simulink model "am_sys1"  (Simulink 3.00)
settings: Solver=ode45  StartTime=0.0  StopTime=999999  MaxStep=0.005  RelTol=1e-3  AbsTol=1e-3
settings Model: SaveTime=off  SaveOutput=off

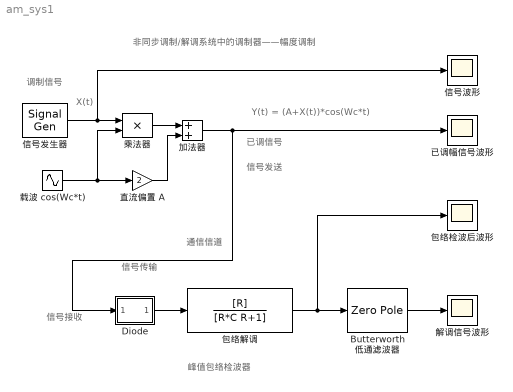
== system am_sys1 ==
  note: 峰值包络检波器
  note: 调制信号
  note: X(t)
  note: Y(t) = (A+X(t))*cos(Wc*t)
  note: 已调信号
  note: 信号发送
  note: 通信信道
  note: 信号传输
  note: 信号接收
  note: 非同步调制/解调系统中的调制器——幅度调制
  Butterworth 低通滤波器 : ZeroPole  Zeros=z  Poles=p  Gain=k  mask(buttap){@1=5*2*pi, @2=4}
      mask prompts: @1 "Cutoff frequency (rad/sec)"; @2 "Order"
      mask help:
      | Analog Butterworth low pass filter.
      |
      | (Requires Signal Processing Toolbox)
      mask init:
      | [z,p,k]=buttap(@2); z=@1*z; p=@1*p; k=real(prod(-p)); [num,den]=zp2tf(z,p,k); w=logspace(log10(@1/10),log10(10*@1),20); h=freqs(num,den,w);
      mask Help: Butterworth low pass filter using MATLAB's butter command.
      mask Display: plot(20*log10(w),20*log10(abs(h)))
  Diode : Subsystem
      mask Type: 二极管
      mask Description: 二极管
      mask Display: plot([0 2 2 2],[0 0 2 -2],[2 4],[2 0],[2 4],[-2 0],[4 4 4 6],[-2 2 0 0]);
  包络检波后波形 : Scope
      settings: TimeRange=1.000000  YMin=-1  YMax=1  SaveToWorkspace=off  SaveName=ScopeData  DataFormat=Matrix
  包络解调 : TransferFcn  Numerator=[R]  Denominator=[R*C R+1]  mask(单元6){@1=1, @2=0.1}
      mask prompts: @1 "电阻值（欧）："; @2 "电容值（法）："
      mask help: 单元6
      mask init:
      | R=@1;C=@2;
      mask Display: plot([0 15],[2 2],[8 8 6 10],[2 0 0 0],[6 10],[-1 -1],[8 8 7 9],[-1 -4 -4 -4],[12.5 12.5 12 13],[2 1 1 1],[12 12],[1 -3],[13 13],[1 -3],[12 13 12.5 12.5],[-3 -3 -3 -4],[12 13],[-4 -4]);
  乘法器 : Product  Inputs=2  SaturateOnIntegerOverflow=on
      mask Type: 乘法器
      mask Description: 乘法器
      mask Display: plot([0 1],[1 0],[0 1],[0 1]);
  加法器 : Sum  Inputs=++  SaturateOnIntegerOverflow=on
  解调信号波形 : Scope
      settings: TimeRange=1.000000  YMin=-0.5  YMax=0.5  SaveToWorkspace=off  SaveName=ScopeData  DataFormat=Matrix
  信号波形 : Scope
      settings: TimeRange=1.000000  YMin=-3  YMax=3  SaveToWorkspace=off  SaveName=ScopeData  DataFormat=Matrix
  信号发生器 : SignalGenerator  WaveForm=sine  Amplitude=1.000000  Frequency=30.000000  Units=rad/sec
  已调幅信号波形 : Scope
      settings: TimeRange=1.000000  YMin=-3  YMax=3  SaveToWorkspace=off  SaveName=ScopeData  DataFormat=Matrix
  载波 cos(Wc*t) : Sin  Amplitude=1  Frequency=F*2*pi  Phase=0  SampleTime=0.005  mask(载波){@1=50}
      mask prompts: @1 "载波频率（Hz）："
      mask help: 载波
      mask init:
      | F=@1;
  直流偏置 A : Gain  Gain=2  SaturateOnIntegerOverflow=on
  wires:
  Butterworth 低通滤波器/1 -> 解调信号波形/1
  信号发生器/1 -> 乘法器/1, 信号波形/1
  Diode/1(out_1) -> 包络解调/1
  加法器/1 -> 已调幅信号波形/1, Diode/1(in_1)
  直流偏置 A/1 -> 加法器/2
  载波 cos(Wc*t)/1 -> 乘法器/2, 直流偏置 A/1
  乘法器/1 -> 加法器/1
  包络解调/1 -> Butterworth 低通滤波器/1, 包络检波后波形/1

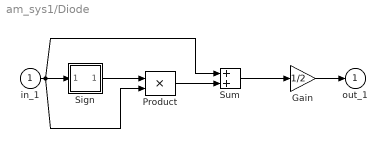
== system am_sys1/Diode ==
  in_1 : Inport  Port=1  PortWidth=-1  SampleTime=-1  DataType=auto
      settings: SignalType=auto
  Gain : Gain  Gain=1/2  SaturateOnIntegerOverflow=on
  Product : Product  Inputs=2  SaturateOnIntegerOverflow=on
  Sign : Subsystem
      mask Type: Sign
      mask Description: y = sign(x)
      mask Help: Sign Function:\n\t\t\ty = 1 if x > 0\n\t\t\ty = 0 if x = 0\n\t\t\ty = -1 if x < 0
      mask Display: plot(-50,-50,50,50,[-50,50],[0,0],[0,0],[-50,50],[-40,0],[-30,-30],[0,40],[30,30])
  Sum : Sum  Inputs=++  SaturateOnIntegerOverflow=on
  out_1 : Outport  Port=1
  wires:
  Sum/1 -> Gain/1
  Product/1 -> Sum/2
  in_1/1 -> Sum/1, Product/2, Sign/1(in_1)
  Sign/1(out_1) -> Product/1
  Gain/1 -> out_1/1

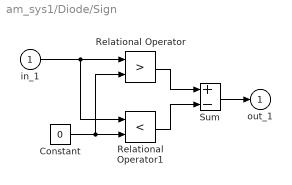
== system am_sys1/Diode/Sign ==
  in_1 : Inport  Port=1  PortWidth=-1  SampleTime=-1  DataType=auto
      settings: SignalType=auto
  Constant : Constant  Value=0
  Relational Operator : RelationalOperator  Operator=>
  Relational Operator1 : RelationalOperator  Operator=<
  Sum : Sum  Inputs=+-  SaturateOnIntegerOverflow=on
  out_1 : Outport  Port=1
  wires:
  in_1/1 -> Relational Operator/1, Relational Operator1/1
  Constant/1 -> Relational Operator1/2, Relational Operator/2
  Relational Operator1/1 -> Sum/2
  Relational Operator/1 -> Sum/1
  Sum/1 -> out_1/1
